simulink model "FIR_filterTest"  (R2019a)
settings: Solver=VariableStepAuto  StartTime=0.0  StopTime=(nSamp +1)*Ts  RelTol=1e-3
InitFcn:
  | FIR_filterTestm;
StopFcn:
  | HPF_Sim = out.HPF_Sim.signals.values(:, 1:FFT_size);
  | HPF_Sim = HPF_Sim(3:8, 1:FFT_size);
  | HPF_Model = HPF_Model(3:8, 1:FFT_size);
  | 
  | filtTestStop;
values from neighbouring files (symbols this model uses):
  FFT_size = 64    [FIR_filterTestm.m]    (also in JMAP_INIT.m; blockVerification.m; block_verScript.m; ksi_verScript.m)
  Ts = 1/Fs    (= 2.08333333333e-05)    [FIR_filterTestm.m]    (also in JMAP_INIT.m; blockVerification.m; block_verScript.m; ksi_verScript.m)
libraries: hdlsllib x2, dsphdlfiltering x2
settings Model: Creator=Showi  LastModifiedBy=Showi

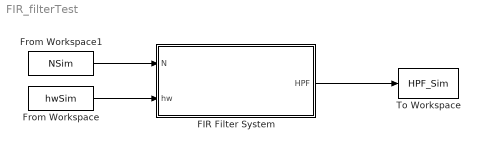
== system FIR_filterTest ==
  FIR Filter System : Subsystem
  From Workspace : FromWorkspace  VariableName=hwSim  SampleTime=Ts
  From Workspace1 : FromWorkspace  VariableName=NSim  SampleTime=Ts
  To Workspace : ToWorkspace  VariableName=HPF_Sim  SaveFormat=Structure With Time  SampleTime=-1
  wires:
  From Workspace1/1 -> FIR Filter System/1(N)
  From Workspace/1 -> FIR Filter System/2(hw)
  FIR Filter System/1(HPF) -> To Workspace/1

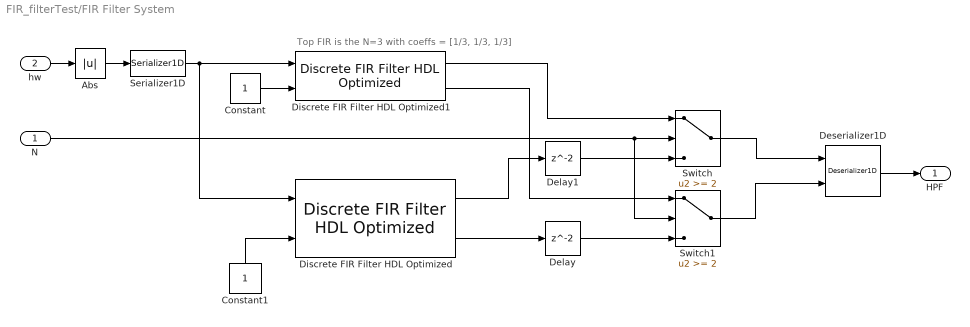
== system FIR_filterTest/FIR Filter System ==
  note: Top FIR is the N=3 with coeffs = [1/3, 1/3, 1/3]
  N : Inport
  hw : Inport  Port=2
  Abs : Abs
  Constant : Constant  OutDataTypeStr=boolean  SampleTime=Ts
  Constant1 : Constant  OutDataTypeStr=boolean  SampleTime=Ts
  Delay : Delay
  Delay1 : Delay
  Deserializer1D : hdlsllib/HDL Operations/Deserializer1D  Ratio=FFT_size  IdleCycles=0  InitialCondition=0  startIn=off  validIn=on  validOut=off  inputDataDimensions=-1  inputSampleTime=-1  inputSignalType=auto
      settings: SourceProductName=Simulink  SourceProductBaseCode=SL
  Discrete FIR Filter HDL Optimized : dsphdlfiltering/Discrete FIR Filter HDL Optimized  NumeratorSource=Property  Numerator=[1]  NumeratorPrototype=[ 0.5, 0.5 ]  FilterStructure=Direct form systolic  SerializationOption=Minimum number of cycles between valid input samples  NumberOfCycles=2  NumberOfMultipliers=2  SimulateUsing=Code generation  roundingMode=Floor  overflowMode=off  CoefficientsDataTypeStr=Inherit: Same word length as input  CoefficientsMin=[]  CoefficientsMax=[]  OutputMin=[]  OutputMax=[]  ResetInputPort=off  HDLGlobalReset=off
      settings: SourceProductName=DSP System Toolbox  SourceProductBaseCode=DS
  Discrete FIR Filter HDL Optimized1 : dsphdlfiltering/Discrete FIR Filter HDL Optimized  NumeratorSource=Property  Numerator=[0.333, 0.333, 0.333]  NumeratorPrototype=[ 0.5, 0.5 ]  FilterStructure=Direct form systolic  SerializationOption=Minimum number of cycles between valid input samples  NumberOfCycles=2  NumberOfMultipliers=2  SimulateUsing=Code generation  roundingMode=Floor  overflowMode=off  CoefficientsDataTypeStr=Inherit: Same word length as input  CoefficientsMin=[]  CoefficientsMax=[]  OutputMin=[]  OutputMax=[]  ResetInputPort=off  HDLGlobalReset=off
      settings: SourceProductName=DSP System Toolbox  SourceProductBaseCode=DS
  Serializer1D : hdlsllib/HDL Operations/Serializer1D  Ratio=FFT_size  IdleCycles=0  validIn=off  startOut=off  validOut=off  inputDataDimensions=-1  inputSampleTime=-1  inputSignalType=auto
      settings: SourceProductName=Simulink  SourceProductBaseCode=SL
  Switch : Switch  Threshold=2
  Switch1 : Switch  Threshold=2
  HPF : Outport
  wires:
  hw/1 -> Abs/1
  Discrete FIR Filter HDL Optimized1/2 -> Switch1/1
  Abs/1 -> Serializer1D/1
  Switch/1 -> Deserializer1D/1
  Deserializer1D/1 -> HPF/1
  N/1 -> Switch1/2, Switch/2
  Discrete FIR Filter HDL Optimized1/1 -> Switch/1
  Discrete FIR Filter HDL Optimized/2 -> Delay/1
  Discrete FIR Filter HDL Optimized/1 -> Delay1/1
  Delay/1 -> Switch1/3
  Switch1/1 -> Deserializer1D/2
  Constant/1 -> Discrete FIR Filter HDL Optimized1/2
  Constant1/1 -> Discrete FIR Filter HDL Optimized/2
  Serializer1D/1 -> Discrete FIR Filter HDL Optimized/1, Discrete FIR Filter HDL Optimized1/1
  Delay1/1 -> Switch/3
